simulink model "car_airdrag"  (R2020b)
settings: Solver=VariableStepAuto  StartTime=0.0  StopTime=2  RelTol=1e-3
settings Model: Creator=kjartan  LastModifiedBy=kjartan

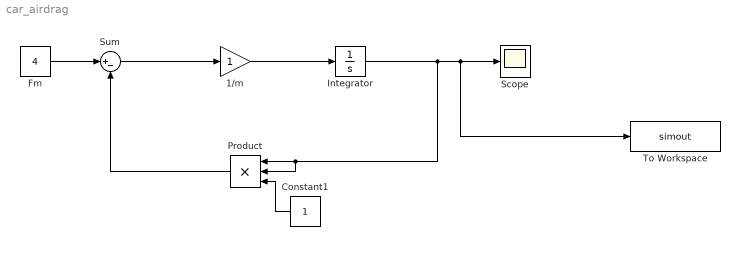
== system car_airdrag ==
  1/m : Gain
  Constant1 : Constant
  Fm : Constant  Value=4
  Integrator : Integrator
  Product : Product  Inputs=3
  Scope : Scope
  Sum : Sum  Inputs=|+-
  To Workspace : ToWorkspace  VariableName=simout  SaveFormat=Timeseries  SampleTime=-1
  wires:
  Integrator/1 -> Product/2, Product/1, To Workspace/1, Scope/1
  Constant1/1 -> Product/3
  Product/1 -> Sum/2
  Fm/1 -> Sum/1
  Sum/1 -> 1/m/1
  1/m/1 -> Integrator/1
